simulink model "NarwhaleSimscape"  (R2021b)
settings: Solver=VariableStepAuto  StartTime=0.0  StopTime=12  FixedStep=10^-3  RelTol=1e-3
undefined symbols (not defined in the file): X, Y, Z
libraries: nesl_utility x34, sm_lib x28, slpidlib x5
(part 2 of 3)

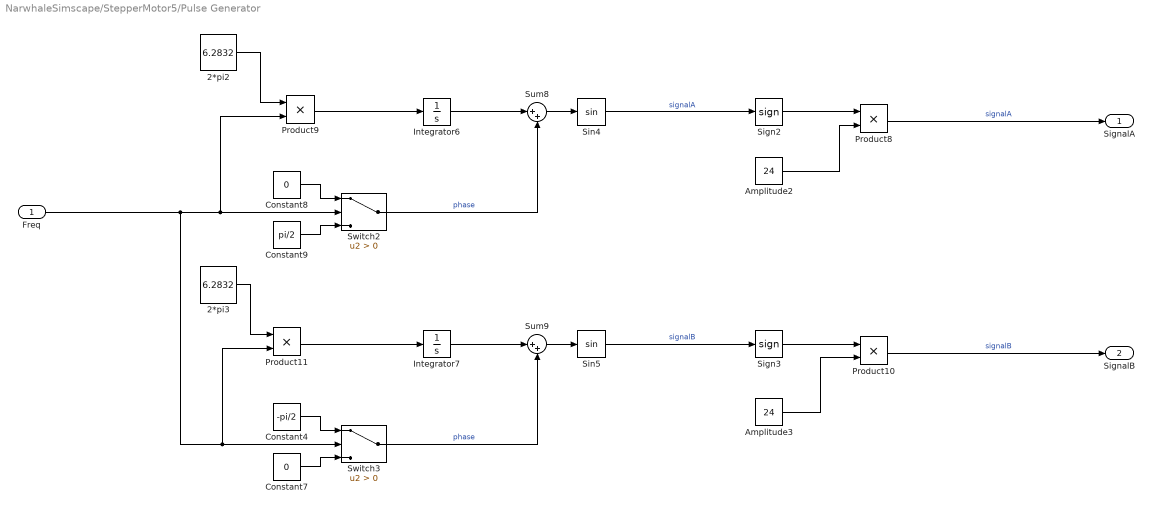
== system NarwhaleSimscape/StepperMotor5/Pulse Generator ==
  Freq : Inport
  2*pi2 : Constant  Value=6.2832
  2*pi3 : Constant  Value=6.2832
  Amplitude2 : Constant  Value=24
  Amplitude3 : Constant  Value=24
  Constant4 : Constant  Value=-pi/2
  Constant7 : Constant  Value=0
  Constant8 : Constant  Value=0
  Constant9 : Constant  Value=pi/2
  Integrator6 : Integrator
  Integrator7 : Integrator
  Product{8..11} (4 alike) : Product
  Sign2 : Signum
  Sign3 : Signum
  Sin4 : Trigonometry
  Sin5 : Trigonometry
  Sum8 : Sum  Inputs=|++
  Sum9 : Sum  Inputs=|++
  Switch2 : Switch  Criteria=u2 > Threshold
  Switch3 : Switch  Criteria=u2 > Threshold
  SignalA : Outport
  SignalB : Outport  Port=2
  wires:
  Product11/1 -> Integrator7/1
  Switch3/1 -> Sum9/2  "phase"
  Sum8/1 -> Sin4/1
  Sign3/1 -> Product10/1
  Integrator7/1 -> Sum9/1
  Freq/1 -> Product11/2, Switch3/2, Product9/2, Switch2/2
  Sin5/1 -> Sign3/1  "signalB"
  Sign2/1 -> Product8/1
  Product10/1 -> SignalB/1  "signalB"
  Product8/1 -> SignalA/1  "signalA"
  Amplitude3/1 -> Product10/2
  Sum9/1 -> Sin5/1
  Amplitude2/1 -> Product8/2
  Integrator6/1 -> Sum8/1
  Constant4/1 -> Switch3/1
  Constant7/1 -> Switch3/3
  2*pi3/1 -> Product11/1
  Switch2/1 -> Sum8/2  "phase"
  Constant9/1 -> Switch2/3
  Constant8/1 -> Switch2/1
  2*pi2/1 -> Product9/1
  Sin4/1 -> Sign2/1  "signalA"
  Product9/1 -> Integrator6/1

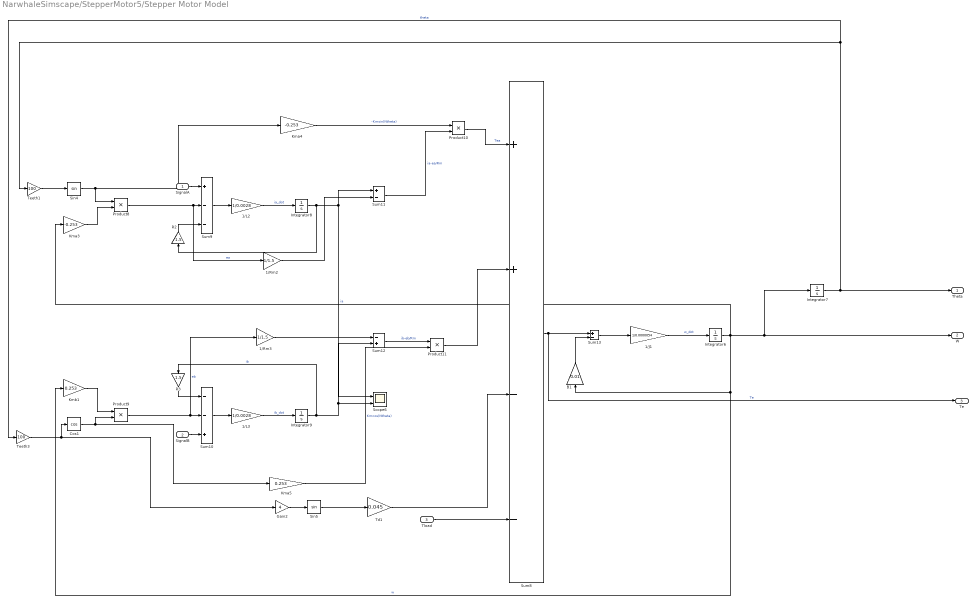
== system NarwhaleSimscape/StepperMotor5/Stepper Motor Model ==
  SignalA : Inport
  SignalB : Inport  Port=2
  Tload : Inport  Port=3
  1/J1 : Gain  Gain=1/0.0000054
  1/L2 : Gain  Gain=1/0.0028
  1/L3 : Gain  Gain=1/0.0028
  1/Rm2 : Gain  Gain=1/1.5
  1/Rm3 : Gain  Gain=1/1.5
  B1 : Gain  Gain=0.01
  Cos1 : Trigonometry  Operator=cos
  Gain2 : Gain  Gain=4
  Integrator{6..9} (4 alike) : Integrator
  Kma3 : Gain  Gain=-0.253
  Kma4 : Gain  Gain=-0.253
  Kma5 : Gain  Gain=0.253
  Kmb1 : Gain  Gain=0.253
  Product{8..11} (4 alike) : Product
  R2 : Gain  Gain=1.5
  R3 : Gain  Gain=1.5
  Scope6 : Scope  NumInputPorts=2
  Sin4 : Trigonometry
  Sin5 : Trigonometry
  Sum10 : Sum  Inputs=--+
  Sum11 : Sum  Inputs=+-
  Sum12 : Sum  Inputs=-+
  Sum13 : Sum  Inputs=+-
  Sum8 : Sum  Inputs=++--
  Sum9 : Sum  Inputs=+--
  Td1 : Gain  Gain=0.045
  Teeth1 : Gain  Gain=100
  Teeth3 : Gain  Gain=100
  Theta : Outport
  W : Outport  Port=2
  Te : Outport  Port=3
  wires:
  Sum10/1 -> 1/L3/1
  1/L3/1 -> Integrator9/1  "ib_dot"
  Cos1/1 -> Kma5/1, Product9/2
  Tload/1 -> Sum8/4
  Gain2/1 -> Sin5/1
  Sum9/1 -> 1/L2/1
  SignalB/1 -> Sum10/3
  Sum13/1 -> 1/J1/1
  Product8/1 -> 1/Rm2/1, Sum9/2  "ea"
  Product11/1 -> Sum8/2
  Teeth3/1 -> Gain2/1, Cos1/1
  SignalA/1 -> Sum9/1
  Sum11/1 -> Product10/2  "ia-ea/Rm"
  1/Rm3/1 -> Sum12/1
  B1/1 -> Sum13/2
  Integrator7/1 -> Theta/1, Teeth1/1, Teeth3/1  "theta"
  Integrator6/1 -> Kmb1/1, B1/1, Kma3/1, W/1, Integrator7/1  "w"
  Sin4/1 -> Kma4/1, Product8/1
  Integrator8/1 -> Scope6/1, Sum11/1, R2/1  "ia"
  R2/1 -> Sum9/3
  Product9/1 -> 1/Rm3/1, Sum10/2  "eb"
  Kma3/1 -> Product8/2
  Sum12/1 -> Product11/1  "ib-eb/Rm"
  1/Rm2/1 -> Sum11/2
  Kmb1/1 -> Product9/1
  Product10/1 -> Sum8/1  "Tea"
  Integrator9/1 -> Scope6/2, Sum12/2, R3/1  "ib"
  Sum8/1 -> Te/1, Sum13/1  "Te"
  1/J1/1 -> Integrator6/1  "w_dot"
  Kma4/1 -> Product10/1  "-Kmsin(Ntheta)"
  Sin5/1 -> Td1/1
  Kma5/1 -> Product11/2  "Kmcos(Ntheta)"
  1/L2/1 -> Integrator8/1  "ia_dot"
  Teeth1/1 -> Sin4/1
  R3/1 -> Sum10/1
  Td1/1 -> Sum8/3

== matlab function NarwhaleSimscape/NarWhale/MATLAB Function1 ==
  data: chi input; qbar output
function qbar  = IKnarwhale5(chi)
    h1= 275.99/1000; % lasted
    h2= 380/1000;
    l1= 20/1000;
    l2= 380/1000;
    l3= 268.23/1000;
    gammabar= [1 1 -1];
    q1 = atan2(gammabar(1)*chi(2),gammabar(1)*chi(1));
    % RRIK
    r = gammabar(2)*sqrt(chi(1)^2 + chi(2)^2)
    z24 = chi(3)+l3-h1
    x24 = r-l1
    if (sqrt(x24^2+z24^2)<= (l2+h2)) && (sqrt(x24^2+z24^2)>=(l2-h2))

        c2 = (x24^2+z24^2-h2^2-l2^2)/(2*h2*l2)
        s2 = gammabar(3)*sqrt(1-c2^2)
        q2 = (atan2(z24,x24)-atan2(l2*s2,h2+l2*c2))-(pi/2) 
        q3 = atan2(s2,c2)+(pi/2)
    else
        % สั่งเกินระยะแขน เกิดท่าประหลาด
        msg = 'error link range.';
        error(msg)
    end 
    q4 = -q2-q3;
    q5 = chi(4);
    qbar = [q1;q2;q3;q4;q5];
end

== matlab function NarwhaleSimscape/NarWhale/IVK_3chi_dot ==
  data: q input; qv5 input; qv output; chi_dot input
function qv = IVK(q,qv5,chi_dot) %q,qv5,chi_dot  % q,taskspace
% h1= 275.99/1000; % lasted
% h2= 380/1000;
% l1= 20.01/1000;
% l2= 380/1000;
% l3= 235/1000;
% h1= 275.99/1000; % lasted
h2= 380/1000;
l1= 20/1000;
l2= 380/1000;
l3= 268.23/1000;

% qv = [                                                                                                                                                                                                                                                                                                                                                                                                                                                                                                                                                                                                                                                                                                                                                                                                                                                                                                                                                                                                                                                                                                                                                                                                                                                                                                                                                                                                                                                                                                                                                                                                                                                                                                                                                                                                                                                                                                                                                                                                                                                                                                                                                                                                                                                                                                                                                                                                                                                                                                                                                                                                                                                                                                                                                                                                                                                                                                                                                                                                                                                                                                                                                                                                                                                                                                                                                                                                                                                                                                                                                                                                                                                                                                                                                                                                                                                                                                                                                                                                                                                                                                                                                                                                                                                                                                                                                                                                                                                                                                                                                                                                                                                                                                                                                                                                                                                                                                                                                                                                                                                                                                                                                                                                                                                                                                                                                                                                                                                                                                                                                                                                                                                                                                                                                                                                                                                                                                                                                                                                                                                                                                                                                                                                                                                                                                                                                                                                                                                                                                                                                                                                                                                                                       (taskspace(4)*cos(q(1)) - taskspace(3)*sin(q(1)))/(l1 + l2*cos(q(2) + q(3)) - 1.0*h2*sin(q(2)) + l3*sin(q(2) + q(3) + q(4)));
%                                                                                                                                                                                                                                                                                                                                                                                                                                                                                                                                                                                                                                                                                                                                                                                                                                                                                                                                                                                                                                                                                                                                                                                                                                                                                                                                                                                                                                                                                                                                                                                                                                                                                                                                                                                                                                                                                                                                                                                                                                                                                                                                                                                                                                                                                                                                                                                                                                                                                                                                                                                                                                                                                                                                                                                                                                                                                                                                                                                                                                                                                                                                                                     -(1.0*(l3^2*taskspace(2)*sin(q(2) + q(3) + q(4))^3*sin(q(2) + q(3))*sin(q(1))^3 + l1*taskspace(3)*cos(q(2) + q(3) + q(4))*cos(q(2) + q(3))*cos(q(1))^2 + l1*taskspace(5)*cos(q(2) + q(3) + q(4))*sin(q(2) + q(3))*cos(q(1))^3 + l2*taskspace(3)*cos(q(2) + q(3) + q(4))*cos(q(2) + q(3))^2*cos(q(1))^2 + l3*taskspace(3)*sin(q(2) + q(3) + q(4))^2*sin(q(2) + q(3))*sin(q(1))^2 + l1*l3*taskspace(1)*cos(q(2) + q(3) + q(4))^2*cos(q(2) + q(3))*sin(q(1))^2 - h2*taskspace(3)*cos(q(2) + q(3) + q(4))*cos(q(2) + q(3))*cos(q(1))^2*sin(q(2)) + l2*taskspace(4)*cos(q(2) + q(3) + q(4))*cos(q(2) + q(3))^2*cos(q(1))*sin(q(1)) + l3^2*taskspace(1)*cos(q(2) + q(3) + q(4))^2*sin(q(2) + q(3) + q(4))*cos(q(2) + q(3))*cos(q(1))^2 - h2*taskspace(5)*cos(q(2) + q(3) + q(4))*sin(q(2) + q(3))*cos(q(1))^3*sin(q(2)) + l1*taskspace(5)*cos(q(2) + q(3) + q(4))*sin(q(2) + q(3))*cos(q(1))*sin(q(1))^2 + l3^2*taskspace(1)*cos(q(2) + q(3) + q(4))*sin(q(2) + q(3) + q(4))^2*sin(q(2) + q(3))*cos(q(1))^2 + l3^2*taskspace(1)*cos(q(2) + q(3) + q(4))^2*sin(q(2) + q(3) + q(4))*cos(q(2) + q(3))*sin(q(1))^2 + l3^2*taskspace(2)*cos(q(2) + q(3) + q(4))*sin(q(2) + q(3) + q(4))^2*cos(q(2) + q(3))*sin(q(1))^3 + l1*l3*taskspace(2)*sin(q(2) + q(3) + q(4))^2*sin(q(2) + q(3))*sin(q(1))^3 - l3*taskspace(4)*sin(q(2) + q(3) + q(4))^2*sin(q(2) + q(3))*cos(q(1))*sin(q(1)) + l3^2*taskspace(1)*cos(q(2) + q(3) + q(4))*sin(q(2) + q(3) + q(4))^2*sin(q(2) + q(3))*sin(q(1))^2 + l3*taskspace(3)*cos(q(2) + q(3) + q(4))*sin(q(2) + q(3) + q(4))*cos(q(2) + q(3))*cos(q(1))^2 + l2*l3*taskspace(1)*cos(q(2) + q(3) + q(4))^2*cos(q(2) + q(3))^2*cos(q(1))^2 + l3*taskspace(3)*cos(q(2) + q(3) + q(4))*sin(q(2) + q(3) + q(4))*cos(q(2) + q(3))*sin(q(1))^2 + l3*taskspace(5)*cos(q(2) + q(3) + q(4))*sin(q(2) + q(3) + q(4))*sin(q(2) + q(3))*cos(q(1))^3 + l2*l3*taskspace(1)*cos(q(2) + q(3) + q(4))^2*cos(q(2) + q(3))^2*sin(q(1))^2 + l1*taskspace(4)*cos(q(2) + q(3) + q(4))*cos(q(2) + q(3))*cos(q(1))*sin(q(1)) + l2*taskspace(5)*cos(q(2) + q(3) + q(4))*cos(q(2) + q(3))*sin(q(2) + q(3))*cos(q(1))^3 + l3^2*taskspace(2)*sin(q(2) + q(3) + q(4))^3*sin(q(2) + q(3))*cos(q(1))^2*sin(q(1)) + l1*l3*taskspace(1)*cos(q(2) + q(3) + q(4))^2*cos(q(2) + q(3))*cos(q(1))^2 + l1*l3*taskspace(2)*sin(q(2) + q(3) + q(4))^2*sin(q(2) + q(3))*cos(q(1))^2*sin(q(1)) - h2*taskspace(5)*cos(q(2) + q(3) + q(4))*sin(q(2) + q(3))*cos(q(1))*sin(q(1))^2*sin(q(2)) - h2*l3*taskspace(2)*sin(q(2) + q(3) + q(4))^2*sin(q(2) + q(3))*sin(q(1))^3*sin(q(2)) + l2*l3*taskspace(2)*cos(q(2) + q(3) + q(4))*sin(q(2) + q(3) + q(4))*cos(q(2) + q(3))^2*sin(q(1))^3 + l3*taskspace(5)*cos(q(2) + q(3) + q(4))*sin(q(2) + q(3) + q(4))*sin(q(2) + q(3))*cos(q(1))*sin(q(1))^2 - h2*taskspace(4)*cos(q(2) + q(3) + q(4))*cos(q(2) + q(3))*cos(q(1))*sin(q(1))*sin(q(2)) + l2*taskspace(5)*cos(q(2) + q(3) + q(4))*cos(q(2) + q(3))*sin(q(2) + q(3))*cos(q(1))*sin(q(1))^2 + l2*l3*taskspace(2)*sin(q(2) + q(3) + q(4))^2*cos(q(2) + q(3))*sin(q(2) + q(3))*sin(q(1))^3 + l1*l3*taskspace(1)*cos(q(2) + q(3) + q(4))*sin(q(2) + q(3) + q(4))*sin(q(2) + q(3))*cos(q(1))^2 + l1*l3*taskspace(2)*cos(q(2) + q(3) + q(4))*sin(q(2) + q(3) + q(4))*cos(q(2) + q(3))*sin(q(1))^3 - h2*l3*taskspace(1)*cos(q(2) + q(3) + q(4))^2*cos(q(2) + q(3))*cos(q(1))^2*sin(q(2)) + l1*l3*taskspace(1)*cos(q(2) + q(3) + q(4))*sin(q(2) + q(3) + q(4))*sin(q(2) + q(3))*sin(q(1))^2 - h2*l3*taskspace(1)*cos(q(2) + q(3) + q(4))^2*cos(q(2) + q(3))*sin(q(1))^2*sin(q(2)) + l3^2*taskspace(2)*cos(q(2) + q(3) + q(4))*sin(q(2) + q(3) + q(4))^2*cos(q(2) + q(3))*cos(q(1))^2*sin(q(1)) + l2*l3*taskspace(2)*cos(q(2) + q(3) + q(4))*sin(q(2) + q(3) + q(4))*cos(q(2) + q(3))^2*cos(q(1))^2*sin(q(1)) + l2*l3*taskspace(1)*cos(q(2) + q(3) + q(4))*sin(q(2) + q(3) + q(4))*cos(q(2) + q(3))*sin(q(2) + q(3))*cos(q(1))^2 + l2*l3*taskspace(1)*cos(q(2) + q(3) + q(4))*sin(q(2) + q(3) + q(4))*cos(q(2) + q(3))*sin(q(2) + q(3))*sin(q(1))^2 + l2*l3*taskspace(2)*sin(q(2) + q(3) + q(4))^2*cos(q(2) + q(3))*sin(q(2) + q(3))*cos(q(1))^2*sin(q(1)) + l1*l3*taskspace(2)*cos(q(2) + q(3) + q(4))*sin(q(2) + q(3) + q(4))*cos(q(2) + q(3))*cos(q(1))^2*sin(q(1)) - h2*l3*taskspace(1)*cos(q(2) + q(3) + q(4))*sin(q(2) + q(3) + q(4))*sin(q(2) + q(3))*cos(q(1))^2*sin(q(2)) - h2*l3*taskspace(2)*cos(q(2) + q(3) + q(4))*sin(q(2) + q(3) + q(4))*cos(q(2) + q(3))*sin(q(1))^3*sin(q(2)) - h2*l3*taskspace(1)*cos(q(2) + q(3) + q(4))*sin(q(2) + q(3) + q(4))*sin(q(2) + q(3))*sin(q(1))^2*sin(q(2)) - h2*l3*taskspace(2)*sin(q(2) + q(3) + q(4))^2*sin(q(2) + q(3))*cos(q(1))^2*sin(q(1))*sin(q(2)) - h2*l3*taskspace(2)*cos(q(2) + q(3) + q(4))*sin(q(2) + q(3) + q(4))*cos(q(2) + q(3))*cos(q(1))^2*sin(q(1))*sin(q(2))))/(h2*cos(q(1))*cos(q(3))*(0.5*l3*sin(2*q(2) + 2*q(3) + 2*q(4)) + 0.5*l2*cos(2.0*q(2) + 2.0*q(3) + q(4)) + 0.5*h2*sin(q(3) + q(4)) - 0.5*h2*sin(2.0*q(2) + q(3) + q(4)) + 0.5*l2*cos(q(4)) + l1*cos(q(2) + q(3) + q(4))));
% (1.0*(h2^2*taskspace(3)*cos(q(2) + q(3) + q(4))*cos(q(1))^2*sin(q(2))^2 + l2^2*taskspace(3)*cos(q(2) + q(3) + q(4))*cos(q(2) + q(3))^2*cos(q(1))^2 + h2^2*l3*taskspace(1)*cos(q(2) + q(3) + q(4))^2*sin(q(1))^2*sin(q(2))^2 + l2*l3*taskspace(3)*sin(q(2) + q(3) + q(4))^2*sin(q(2) + q(3))*sin(q(1))^2 + l2^2*taskspace(5)*cos(q(2) + q(3) + q(4))*cos(q(2) + q(3))*sin(q(2) + q(3))*cos(q(1))^3 + h2*l3*taskspace(3)*sin(q(2) + q(3) + q(4))^2*cos(q(2))*sin(q(1))^2 + l2^2*taskspace(4)*cos(q(2) + q(3) + q(4))*cos(q(2) + q(3))^2*cos(q(1))*sin(q(1)) + l2*l3^2*taskspace(2)*sin(q(2) + q(3) + q(4))^3*sin(q(2) + q(3))*sin(q(1))^3 + l1*l2*taskspace(3)*cos(q(2) + q(3) + q(4))*cos(q(2) + q(3))*cos(q(1))^2 - 1.0*h2^2*taskspace(5)*cos(q(2) + q(3) + q(4))*cos(q(1))^3*cos(q(2))*sin(q(2)) + h2*l3^2*taskspace(2)*sin(q(2) + q(3) + q(4))^3*cos(q(2))*sin(q(1))^3 + l1*l2*taskspace(5)*cos(q(2) + q(3) + q(4))*sin(q(2) + q(3))*cos(q(1))^3 + h2^2*taskspace(4)*cos(q(2) + q(3) + q(4))*cos(q(1))*sin(q(1))*sin(q(2))^2 + l2^2*l3*taskspace(1)*cos(q(2) + q(3) + q(4))^2*cos(q(2) + q(3))^2*cos(q(1))^2 + h2*l1*taskspace(5)*cos(q(2) + q(3) + q(4))*cos(q(1))^3*cos(q(2)) + l2^2*l3*taskspace(1)*cos(q(2) + q(3) + q(4))^2*cos(q(2) + q(3))^2*sin(q(1))^2 - 1.0*h2*l1*taskspace(3)*cos(q(2) + q(3) + q(4))*cos(q(1))^2*sin(q(2)) + h2^2*l3*taskspace(1)*cos(q(2) + q(3) + q(4))^2*cos(q(1))^2*sin(q(2))^2 - 1.0*h2*l3*taskspace(3)*cos(q(2) + q(3) + q(4))*sin(q(2) + q(3) + q(4))*sin(q(1))^2*sin(q(2)) + l1*l2*taskspace(4)*cos(q(2) + q(3) + q(4))*cos(q(2) + q(3))*cos(q(1))*sin(q(1)) + l2^2*taskspace(5)*cos(q(2) + q(3) + q(4))*cos(q(2) + q(3))*sin(q(2) + q(3))*cos(q(1))*sin(q(1))^2 + l2^2*l3*taskspace(2)*sin(q(2) + q(3) + q(4))^2*cos(q(2) + q(3))*sin(q(2) + q(3))*sin(q(1))^3 - 1.0*h2*l1*taskspace(4)*cos(q(2) + q(3) + q(4))*cos(q(1))*sin(q(1))*sin(q(2)) + l2*l3^2*taskspace(2)*sin(q(2) + q(3) + q(4))^3*sin(q(2) + q(3))*cos(q(1))^2*sin(q(1)) + l1*l2*l3*taskspace(1)*cos(q(2) + q(3) + q(4))^2*cos(q(2) + q(3))*cos(q(1))^2 + h2*l2*taskspace(5)*cos(q(2) + q(3) + q(4))*cos(q(2) + q(3))*cos(q(1))^3*cos(q(2)) + l1*l2*l3*taskspace(1)*cos(q(2) + q(3) + q(4))^2*cos(q(2) + q(3))*sin(q(1))^2 + h2*l3^2*taskspace(2)*sin(q(2) + q(3) + q(4))^3*cos(q(1))^2*cos(q(2))*sin(q(1)) - 2.0*h2*l2*taskspace(3)*cos(q(2) + q(3) + q(4))*cos(q(2) + q(3))*cos(q(1))^2*sin(q(2)) + l2*l3^2*taskspace(1)*cos(q(2) + q(3) + q(4))^2*sin(q(2) + q(3) + q(4))*cos(q(2) + q(3))*cos(q(1))^2 - 1.0*h2^2*taskspace(5)*cos(q(2) + q(3) + q(4))*cos(q(1))*cos(q(2))*sin(q(1))^2*sin(q(2)) - 1.0*h2^2*l3*taskspace(2)*sin(q(2) + q(3) + q(4))^2*cos(q(2))*sin(q(1))^3*sin(q(2)) - 1.0*h2*l2*taskspace(5)*cos(q(2) + q(3) + q(4))*sin(q(2) + q(3))*cos(q(1))^3*sin(q(2)) + l1*l2*taskspace(5)*cos(q(2) + q(3) + q(4))*sin(q(2) + q(3))*cos(q(1))*sin(q(1))^2 + l2*l3^2*taskspace(1)*cos(q(2) + q(3) + q(4))*sin(q(2) + q(3) + q(4))^2*sin(q(2) + q(3))*cos(q(1))^2 + l2*l3^2*taskspace(1)*cos(q(2) + q(3) + q(4))^2*sin(q(2) + q(3) + q(4))*cos(q(2) + q(3))*sin(q(1))^2 + l2*l3^2*taskspace(2)*cos(q(2) + q(3) + q(4))*sin(q(2) + q(3) + q(4))^2*cos(q(2) + q(3))*sin(q(1))^3 + l2^2*l3*taskspace(2)*cos(q(2) + q(3) + q(4))*sin(q(2) + q(3) + q(4))*cos(q(2) + q(3))^2*sin(q(1))^3 + l1*l2*l3*taskspace(2)*sin(q(2) + q(3) + q(4))^2*sin(q(2) + q(3))*sin(q(1))^3 - 1.0*l2*l3*taskspace(4)*sin(q(2) + q(3) + q(4))^2*sin(q(2) + q(3))*cos(q(1))*sin(q(1)) + l2*l3^2*taskspace(1)*cos(q(2) + q(3) + q(4))*sin(q(2) + q(3) + q(4))^2*sin(q(2) + q(3))*sin(q(1))^2 - 1.0*h2*l1*l3*taskspace(1)*cos(q(2) + q(3) + q(4))^2*cos(q(1))^2*sin(q(2)) + h2*l1*taskspace(5)*cos(q(2) + q(3) + q(4))*cos(q(1))*cos(q(2))*sin(q(1))^2 + h2*l3^2*taskspace(1)*cos(q(2) + q(3) + q(4))*sin(q(2) + q(3) + q(4))^2*cos(q(1))^2*cos(q(2)) - 1.0*h2*l1*l3*taskspace(1)*cos(q(2) + q(3) + q(4))^2*sin(q(1))^2*sin(q(2)) + h2*l1*l3*taskspace(2)*sin(q(2) + q(3) + q(4))^2*cos(q(2))*sin(q(1))^3 - 1.0*h2*l3*taskspace(4)*sin(q(2) + q(3) + q(4))^2*cos(q(1))*cos(q(2))*sin(q(1)) + h2*l3^2*taskspace(1)*cos(q(2) + q(3) + q(4))*sin(q(2) + q(3) + q(4))^2*cos(q(2))*sin(q(1))^2 - 1.0*h2*l3^2*taskspace(1)*cos(q(2) + q(3) + q(4))^2*sin(q(2) + q(3) + q(4))*cos(q(1))^2*sin(q(2)) + l2*l3*taskspace(3)*cos(q(2) + q(3) + q(4))*sin(q(2) + q(3) + q(4))*cos(q(2) + q(3))*cos(q(1))^2 - 1.0*h2*l3^2*taskspace(1)*cos(q(2) + q(3) + q(4))^2*sin(q(2) + q(3) + q(4))*sin(q(1))^2*sin(q(2)) - 1.0*h2*l3^2*taskspace(2)*cos(q(2) + q(3) + q(4))*sin(q(2) + q(3) + q(4))^2*sin(q(1))^3*sin(q(2)) + h2^2*l3*taskspace(2)*cos(q(2) + q(3) + q(4))*sin(q(2) + q(3) + q(4))*sin(q(1))^3*sin(q(2))^2 + l2*l3*taskspace(3)*cos(q(2) + q(3) + q(4))*sin(q(2) + q(3) + q(4))*cos(q(2) + q(3))*sin(q(1))^2 + l2*l3*taskspace(5)*cos(q(2) + q(3) + q(4))*sin(q(2) + q(3) + q(4))*sin(q(2) + q(3))*cos(q(1))^3 + h2*l3*taskspace(5)*cos(q(2) + q(3) + q(4))*sin(q(2) + q(3) + q(4))*cos(q(1))^3*cos(q(2)) - 1.0*h2*l3*taskspace(3)*cos(q(2) + q(3) + q(4))*sin(q(2) + q(3) + q(4))*cos(q(1))^2*sin(q(2)) - 2.0*h2*l2*taskspace(4)*cos(q(2) + q(3) + q(4))*cos(q(2) + q(3))*cos(q(1))*sin(q(1))*sin(q(2)) + l2^2*l3*taskspace(2)*sin(q(2) + q(3) + q(4))^2*cos(q(2) + q(3))*sin(q(2) + q(3))*cos(q(1))^2*sin(q(1)) - 1.0*h2^2*l3*taskspace(1)*cos(q(2) + q(3) + q(4))*sin(q(2) + q(3) + q(4))*cos(q(1))^2*cos(q(2))*sin(q(2)) + l1*l2*l3*taskspace(1)*cos(q(2) + q(3) + q(4))*sin(q(2) + q(3) + q(4))*sin(q(2) + q(3))*cos(q(1))^2 + l1*l2*l3*taskspace(2)*cos(q(2) + q(3) + q(4))*sin(q(2) + q(3) + q(4))*cos(q(2) + q(3))*sin(q(1))^3 - 1.0*h2^2*l3*taskspace(1)*cos(q(2) + q(3) + q(4))*sin(q(2) + q(3) + q(4))*cos(q(2))*sin(q(1))^2*sin(q(2)) - 2.0*h2*l2*l3*taskspace(1)*cos(q(2) + q(3) + q(4))^2*cos(q(2) + q(3))*cos(q(1))^2*sin(q(2)) + l1*l2*l3*taskspace(1)*cos(q(2) + q(3) + q(4))*sin(q(2) + q(3) + q(4))*sin(q(2) + q(3))*sin(q(1))^2 + h2*l2*taskspace(5)*cos(q(2) + q(3) + q(4))*cos(q(2) + q(3))*cos(q(1))*cos(q(2))*sin(q(1))^2 - 2.0*h2*l2*l3*taskspace(1)*cos(q(2) + q(3) + q(4))^2*cos(q(2) + q(3))*sin(q(1))^2*sin(q(2)) + h2*l2*l3*taskspace(2)*sin(q(2) + q(3) + q(4))^2*cos(q(2) + q(3))*cos(q(2))*sin(q(1))^3 + h2*l1*l3*taskspace(1)*cos(q(2) + q(3) + q(4))*sin(q(2) + q(3) + q(4))*cos(q(1))^2*cos(q(2)) - 1.0*h2^2*l3*taskspace(2)*sin(q(2) + q(3) + q(4))^2*cos(q(1))^2*cos(q(2))*sin(q(1))*sin(q(2)) + l2*l3^2*taskspace(2)*cos(q(2) + q(3) + q(4))*sin(q(2) + q(3) + q(4))^2*cos(q(2) + q(3))*cos(q(1))^2*sin(q(1)) + l2^2*l3*taskspace(2)*cos(q(2) + q(3) + q(4))*sin(q(2) + q(3) + q(4))*cos(q(2) + q(3))^2*cos(q(1))^2*sin(q(1)) + h2*l1*l3*taskspace(1)*cos(q(2) + q(3) + q(4))*sin(q(2) + q(3) + q(4))*cos(q(2))*sin(q(1))^2 + l1*l2*l3*taskspace(2)*sin(q(2) + q(3) + q(4))^2*sin(q(2) + q(3))*cos(q(1))^2*sin(q(1)) - 1.0*h2*l2*taskspace(5)*cos(q(2) + q(3) + q(4))*sin(q(2) + q(3))*cos(q(1))*sin(q(1))^2*sin(q(2)) - 1.0*h2*l2*l3*taskspace(2)*sin(q(2) + q(3) + q(4))^2*sin(q(2) + q(3))*sin(q(1))^3*sin(q(2)) - 1.0*h2*l1*l3*taskspace(2)*cos(q(2) + q(3) + q(4))*sin(q(2) + q(3) + q(4))*sin(q(1))^3*sin(q(2)) + h2*l1*l3*taskspace(2)*sin(q(2) + q(3) + q(4))^2*cos(q(1))^2*cos(q(2))*sin(q(1)) - 1.0*h2*l3^2*taskspace(2)*cos(q(2) + q(3) + q(4))*sin(q(2) + q(3) + q(4))^2*cos(q(1))^2*sin(q(1))*sin(q(2)) + h2^2*l3*taskspace(2)*cos(q(2) + q(3) + q(4))*sin(q(2) + q(3) + q(4))*cos(q(1))^2*sin(q(1))*sin(q(2))^2 + l2*l3*taskspace(5)*cos(q(2) + q(3) + q(4))*sin(q(2) + q(3) + q(4))*sin(q(2) + q(3))*cos(q(1))*sin(q(1))^2 + h2*l3*taskspace(5)*cos(q(2) + q(3) + q(4))*sin(q(2) + q(3) + q(4))*cos(q(1))*cos(q(2))*sin(q(1))^2 + l2^2*l3*taskspace(1)*cos(q(2) + q(3) + q(4))*sin(q(2) + q(3) + q(4))*cos(q(2) + q(3))*sin(q(2) + q(3))*cos(q(1))^2 + l2^2*l3*taskspace(1)*cos(q(2) + q(3) + q(4))*sin(q(2) + q(3) + q(4))*cos(q(2) + q(3))*sin(q(2) + q(3))*sin(q(1))^2 + h2*l2*l3*taskspace(1)*cos(q(2) + q(3) + q(4))*sin(q(2) + q(3) + q(4))*cos(q(2) + q(3))*cos(q(2))*sin(q(1))^2 + l1*l2*l3*taskspace(2)*cos(q(2) + q(3) + q(4))*sin(q(2) + q(3) + q(4))*cos(q(2) + q(3))*cos(q(1))^2*sin(q(1)) - 1.0*h2*l2*l3*taskspace(1)*cos(q(2) + q(3) + q(4))*sin(q(2) + q(3) + q(4))*sin(q(2) + q(3))*cos(q(1))^2*sin(q(2)) - 2.0*h2*l2*l3*taskspace(2)*cos(q(2) + q(3) + q(4))*sin(q(2) + q(3) + q(4))*cos(q(2) + q(3))*sin(q(1))^3*sin(q(2)) + h2*l2*l3*taskspace(2)*sin(q(2) + q(3) + q(4))^2*cos(q(2) + q(3))*cos(q(1))^2*cos(q(2))*sin(q(1)) - 1.0*h2*l2*l3*taskspace(1)*cos(q(2) + q(3) + q(4))*sin(q(2) + q(3) + q(4))*sin(q(2) + q(3))*sin(q(1))^2*sin(q(2)) - 1.0*h2*l2*l3*taskspace(2)*sin(q(2) + q(3) + q(4))^2*sin(q(2) + q(3))*cos(q(1))^2*sin(q(1))*sin(q(2)) - 1.0*h2*l1*l3*taskspace(2)*cos(q(2) + q(3) + q(4))*sin(q(2) + q(3) + q(4))*cos(q(1))^2*sin(q(1))*sin(q(2)) + h2*l2*l3*taskspace(1)*cos(q(2) + q(3) + q(4))*sin(q(2) + q(3) + q(4))*cos(q(2) + q(3))*cos(q(1))^2*cos(q(2)) - 2.0*h2*l2*l3*taskspace(2)*cos(q(2) + q(3) + q(4))*sin(q(2) + q(3) + q(4))*cos(q(2) + q(3))*cos(q(1))^2*sin(q(1))*sin(q(2))))/(h2*l2*cos(q(1))*cos(q(3))*(0.5*l3*sin(2*q(2) + 2*q(3) + 2*q(4)) + 0.5*l2*cos(2.0*q(2) + 2.0*q(3) + q(4)) + 0.5*h2*sin(q(3) + q(4)) - 0.5*h2*sin(2.0*q(2) + q(3) + q(4)) + 0.5*l2*cos(q(4)) + l1*cos(q(2) + q(3) + q(4))));
%                                                                                                                                                                                                                                                                                                                                                                                                                                                                                                                                                                                                                                                                                                                                                                                                                                                                                                                                                                                                                                                                                                                                                                                     -(1.0*(l3^2*taskspace(2)*sin(q(2) + q(3) + q(4))^3*cos(q(2))*sin(q(1))^3 + l1*taskspace(5)*cos(q(2) + q(3) + q(4))*cos(q(1))^3*cos(q(2)) - l1*taskspace(3)*cos(q(2) + q(3) + q(4))*cos(q(1))^2*sin(q(2)) + h2*taskspace(3)*cos(q(2) + q(3) + q(4))*cos(q(1))^2*sin(q(2))^2 + l3*taskspace(3)*sin(q(2) + q(3) + q(4))^2*cos(q(2))*sin(q(1))^2 + l2*taskspace(5)*cos(q(2) + q(3) + q(4))*cos(q(2) + q(3))*cos(q(1))^3*cos(q(2)) + l3^2*taskspace(2)*sin(q(2) + q(3) + q(4))^3*cos(q(1))^2*cos(q(2))*sin(q(1)) - l2*taskspace(3)*cos(q(2) + q(3) + q(4))*cos(q(2) + q(3))*cos(q(1))^2*sin(q(2)) + l2*taskspace(3)*sin(q(2) + q(3) + q(4))*cos(q(2) + q(3))*cos(q(2))*sin(q(1))^2 - l1*l3*taskspace(1)*cos(q(2) + q(3) + q(4))^2*cos(q(1))^2*sin(q(2)) - h2*taskspace(5)*cos(q(2) + q(3) + q(4))*cos(q(1))^3*cos(q(2))*sin(q(2)) + l1*taskspace(5)*cos(q(2) + q(3) + q(4))*cos(q(1))*cos(q(2))*sin(q(1))^2 + l2*taskspace(3)*sin(q(2) + q(3) + q(4))*sin(q(2) + q(3))*sin(q(1))^2*sin(q(2)) + l3^2*taskspace(1)*cos(q(2) + q(3) + q(4))*sin(q(2) + q(3) + q(4))^2*cos(q(1))^2*cos(q(2)) - l1*l3*taskspace(1)*cos(q(2) + q(3) + q(4))^2*sin(q(1))^2*sin(q(2)) + l1*l3*taskspace(2)*sin(q(2) + q(3) + q(4))^2*cos(q(2))*sin(q(1))^3 + h2*taskspace(4)*cos(q(2) + q(3) + q(4))*cos(q(1))*sin(q(1))*sin(q(2))^2 - l3*taskspace(4)*sin(q(2) + q(3) + q(4))^2*cos(q(1))*cos(q(2))*sin(q(1)) + l3^2*taskspace(1)*cos(q(2) + q(3) + q(4))*sin(q(2) + q(3) + q(4))^2*cos(q(2))*sin(q(1))^2 - l3^2*taskspace(1)*cos(q(2) + q(3) + q(4))^2*sin(q(2) + q(3) + q(4))*cos(q(1))^2*sin(q(2)) - l3^2*taskspace(1)*cos(q(2) + q(3) + q(4))^2*sin(q(2) + q(3) + q(4))*sin(q(1))^2*sin(q(2)) - l3^2*taskspace(2)*cos(q(2) + q(3) + q(4))*sin(q(2) + q(3) + q(4))^2*sin(q(1))^3*sin(q(2)) + l3*taskspace(5)*cos(q(2) + q(3) + q(4))*sin(q(2) + q(3) + q(4))*cos(q(1))^3*cos(q(2)) - l3*taskspace(3)*cos(q(2) + q(3) + q(4))*sin(q(2) + q(3) + q(4))*cos(q(1))^2*sin(q(2)) + h2*l3*taskspace(1)*cos(q(2) + q(3) + q(4))^2*cos(q(1))^2*sin(q(2))^2 - l3*taskspace(3)*cos(q(2) + q(3) + q(4))*sin(q(2) + q(3) + q(4))*sin(q(1))^2*sin(q(2)) + h2*l3*taskspace(1)*cos(q(2) + q(3) + q(4))^2*sin(q(1))^2*sin(q(2))^2 + l2^2*taskspace(1)*cos(q(2) + q(3) + q(4))*cos(q(2) + q(3))^2*cos(q(1))^2*cos(q(2)) + l2^2*taskspace(1)*cos(q(2) + q(3) + q(4))*cos(q(2) + q(3))^2*cos(q(2))*sin(q(1))^2 + l2^2*taskspace(2)*sin(q(2) + q(3) + q(4))*cos(q(2) + q(3))^2*cos(q(2))*sin(q(1))^3 - l1*taskspace(4)*cos(q(2) + q(3) + q(4))*cos(q(1))*sin(q(1))*sin(q(2)) + l1*l3*taskspace(1)*cos(q(2) + q(3) + q(4))*sin(q(2) + q(3) + q(4))*cos(q(2))*sin(q(1))^2 - h2*l2*taskspace(2)*sin(q(2) + q(3) + q(4))*sin(q(2) + q(3))*sin(q(1))^3*sin(q(2))^2 + l2*l3*taskspace(2)*sin(q(2) + q(3) + q(4))^2*sin(q(2) + q(3))*sin(q(1))^3*sin(q(2)) - l1*l3*taskspace(2)*cos(q(2) + q(3) + q(4))*sin(q(2) + q(3) + q(4))*sin(q(1))^3*sin(q(2)) + l1*l3*taskspace(2)*sin(q(2) + q(3) + q(4))^2*cos(q(1))^2*cos(q(2))*sin(q(1)) - h2*taskspace(5)*cos(q(2) + q(3) + q(4))*cos(q(1))*cos(q(2))*sin(q(1))^2*sin(q(2)) + l2^2*taskspace(1)*cos(q(2) + q(3) + q(4))*cos(q(2) + q(3))*sin(q(2) + q(3))*cos(q(1))^2*sin(q(2)) - h2*l3*taskspace(2)*sin(q(2) + q(3) + q(4))^2*cos(q(2))*sin(q(1))^3*sin(q(2)) + l2^2*taskspace(1)*cos(q(2) + q(3) + q(4))*cos(q(2) + q(3))*sin(q(2) + q(3))*sin(q(1))^2*sin(q(2)) - l3^2*taskspace(2)*cos(q(2) + q(3) + q(4))*sin(q(2) + q(3) + q(4))^2*cos(q(1))^2*sin(q(1))*sin(q(2)) + l2^2*taskspace(2)*sin(q(2) + q(3) + q(4))*cos(q(2) + q(3))*sin(q(2) + q(3))*sin(q(1))^3*sin(q(2)) + l3*taskspace(5)*cos(q(2) + q(3) + q(4))*sin(q(2) + q(3) + q(4))*cos(q(1))*cos(q(2))*sin(q(1))^2 + h2*l3*taskspace(2)*cos(q(2) + q(3) + q(4))*sin(q(2) + q(3) + q(4))*sin(q(1))^3*sin(q(2))^2 + l1*l2*taskspace(1)*cos(q(2) + q(3) + q(4))*cos(q(2) + q(3))*cos(q(1))^2*cos(q(2)) + l1*l2*taskspace(1)*cos(q(2) + q(3) + q(4))*cos(q(2) + q(3))*cos(q(2))*sin(q(1))^2 + l1*l2*taskspace(1)*cos(q(2) + q(3) + q(4))*sin(q(2) + q(3))*cos(q(1))^2*sin(q(2)) + l1*l2*taskspace(2)*sin(q(2) + q(3) + q(4))*cos(q(2) + q(3))*cos(q(2))*sin(q(1))^3 - l2*taskspace(4)*cos(q(2) + q(3) + q(4))*cos(q(2) + q(3))*cos(q(1))*sin(q(1))*sin(q(2)) - l2*taskspace(4)*sin(q(2) + q(3) + q(4))*cos(q(2) + q(3))*cos(q(1))*cos(q(2))*sin(q(1)) + l1*l2*taskspace(1)*cos(q(2) + q(3) + q(4))*sin(q(2) + q(3))*sin(q(1))^2*sin(q(2)) + l1*l2*taskspace(2)*sin(q(2) + q(3) + q(4))*sin(q(2) + q(3))*sin(q(1))^3*sin(q(2)) + l2^2*taskspace(2)*sin(q(2) + q(3) + q(4))*cos(q(2) + q(3))^2*cos(q(1))^2*cos(q(2))*sin(q(1)) - l2*taskspace(4)*sin(q(2) + q(3) + q(4))*sin(q(2) + q(3))*cos(q(1))*sin(q(1))*sin(q(2)) - l2*l3*taskspace(1)*cos(q(2) + q(3) + q(4))^2*cos(q(2) + q(3))*cos(q(1))^2*sin(q(2)) + l2*taskspace(5)*cos(q(2) + q(3) + q(4))*cos(q(2) + q(3))*cos(q(1))*cos(q(2))*sin(q(1))^2 - h2*l2*taskspace(1)*cos(q(2) + q(3) + q(4))*sin(q(2) + q(3))*cos(q(1))^2*sin(q(2))^2 - l2*l3*taskspace(1)*cos(q(2) + q(3) + q(4))^2*cos(q(2) + q(3))*sin(q(1))^2*sin(q(2)) + 2.0*l2*l3*taskspace(2)*sin(q(2) + q(3) + q(4))^2*cos(q(2) + q(3))*cos(q(2))*sin(q(1))^3 + l1*l3*taskspace(1)*cos(q(2) + q(3) + q(4))*sin(q(2) + q(3) + q(4))*cos(q(1))^2*cos(q(2)) - h2*l2*taskspace(1)*cos(q(2) + q(3) + q(4))*sin(q(2) + q(3))*sin(q(1))^2*sin(q(2))^2 - h2*l3*taskspace(2)*sin(q(2) + q(3) + q(4))^2*cos(q(1))^2*cos(q(2))*sin(q(1))*sin(q(2)) + l2^2*taskspace(2)*sin(q(2) + q(3) + q(4))*cos(q(2) + q(3))*sin(q(2) + q(3))*cos(q(1))^2*sin(q(1))*sin(q(2)) + h2*l3*taskspace(2)*cos(q(2) + q(3) + q(4))*sin(q(2) + q(3) + q(4))*cos(q(1))^2*sin(q(1))*sin(q(2))^2 - h2*l2*taskspace(1)*cos(q(2) + q(3) + q(4))*cos(q(2) + q(3))*cos(q(1))^2*cos(q(2))*sin(q(2)) - h2*l2*taskspace(1)*cos(q(2) + q(3) + q(4))*cos(q(2) + q(3))*cos(q(2))*sin(q(1))^2*sin(q(2)) + l1*l2*taskspace(2)*sin(q(2) + q(3) + q(4))*cos(q(2) + q(3))*cos(q(1))^2*cos(q(2))*sin(q(1)) - h2*l2*taskspace(2)*sin(q(2) + q(3) + q(4))*cos(q(2) + q(3))*cos(q(2))*sin(q(1))^3*sin(q(2)) + l1*l2*taskspace(2)*sin(q(2) + q(3) + q(4))*sin(q(2) + q(3))*cos(q(1))^2*sin(q(1))*sin(q(2)) + 2.0*l2*l3*taskspace(1)*cos(q(2) + q(3) + q(4))*sin(q(2) + q(3) + q(4))*cos(q(2) + q(3))*cos(q(1))^2*cos(q(2)) + 2.0*l2*l3*taskspace(1)*cos(q(2) + q(3) + q(4))*sin(q(2) + q(3) + q(4))*cos(q(2) + q(3))*cos(q(2))*sin(q(1))^2 + l2*l3*taskspace(1)*cos(q(2) + q(3) + q(4))*sin(q(2) + q(3) + q(4))*sin(q(2) + q(3))*cos(q(1))^2*sin(q(2)) - l2*l3*taskspace(2)*cos(q(2) + q(3) + q(4))*sin(q(2) + q(3) + q(4))*cos(q(2) + q(3))*sin(q(1))^3*sin(q(2)) + 2.0*l2*l3*taskspace(2)*sin(q(2) + q(3) + q(4))^2*cos(q(2) + q(3))*cos(q(1))^2*cos(q(2))*sin(q(1)) + l2*l3*taskspace(1)*cos(q(2) + q(3) + q(4))*sin(q(2) + q(3) + q(4))*sin(q(2) + q(3))*sin(q(1))^2*sin(q(2)) - h2*l3*taskspace(1)*cos(q(2) + q(3) + q(4))*sin(q(2) + q(3) + q(4))*cos(q(1))^2*cos(q(2))*sin(q(2)) - h2*l2*taskspace(2)*sin(q(2) + q(3) + q(4))*sin(q(2) + q(3))*cos(q(1))^2*sin(q(1))*sin(q(2))^2 - h2*l3*taskspace(1)*cos(q(2) + q(3) + q(4))*sin(q(2) + q(3) + q(4))*cos(q(2))*sin(q(1))^2*sin(q(2)) + l2*l3*taskspace(2)*sin(q(2) + q(3) + q(4))^2*sin(q(2) + q(3))*cos(q(1))^2*sin(q(1))*sin(q(2)) - l1*l3*taskspace(2)*cos(q(2) + q(3) + q(4))*sin(q(2) + q(3) + q(4))*cos(q(1))^2*sin(q(1))*sin(q(2)) - h2*l2*taskspace(2)*sin(q(2) + q(3) + q(4))*cos(q(2) + q(3))*cos(q(1))^2*cos(q(2))*sin(q(1))*sin(q(2)) - l2*l3*taskspace(2)*cos(q(2) + q(3) + q(4))*sin(q(2) + q(3) + q(4))*cos(q(2) + q(3))*cos(q(1))^2*sin(q(1))*sin(q(2))))/(l2*cos(q(1))*cos(q(3))*(0.5*l3*sin(2*q(2) + 2*q(3) + 2*q(4)) + 0.5*l2*cos(2.0*q(2) + 2.0*q(3) + q(4)) + 0.5*h2*sin(q(3) + q(4)) - 0.5*h2*sin(2.0*q(2) + q(3) + q(4)) + 0.5*l2*cos(q(4)) + l1*cos(q(2) + q(3) + q(4))));
%                                                                                                                                                                                                                                                                                                                                                                                                                                                                                                                                                                                                                                                                                                                                                                                                                                                                                                                                                                                                                                                                                                                                                                                                                                                                                                                                                                                                                                                                                                                                                                                                                                                                                                                                                                                                                                                                                                                                                                                                                                                                                                                                                                                                                                                                                                                                                                                                                                                                                                                                                                                                                                                                                                                                                                                                                                                                                                                                                                                                                                                                                                                                                                                                                                                                                                                                                                                                                                                                                                                                                                                                                                                                                                                                                                                                                                                                                                                                                                                                                                                                                                                                                                                                                                                                                                                                                                                                                                                                                                                                                                                                                                                                                                                                                                                                                                                                                                                                                                                                                                                                                                                                                                                                                                                                                                                                                                                                                                                                                                                                                                                                                                                                                                                                                                                                                                                                                                                                                                                                                                                                                                                                                                                                                                                                                                                                                                                                                                                                                               -(1.0*(l1*taskspace(2) - 1.0*taskspace(4)*cos(q(1)) + taskspace(3)*sin(q(1)) - 1.0*h2*taskspace(2)*sin(q(2)) + 1.0*l3*taskspace(2)*sin(q(2) + q(3) + q(4)) + 1.0*l2*taskspace(2)*cos(q(2) + q(3))))/(0.5*l3*sin(2*q(2) + 2*q(3) + 2*q(4)) - 0.5*h2*sin(2*q(2) + q(3) + q(4)) + 0.5*h2*sin(q(3) + q(4)) + 0.5*l2*cos(q(4)) + 0.5*l2*cos(2*q(2) + 2*q(3) + q(4)) + 1.0*l1*cos(q(2) + q(3) + q(4)))]
%  
% 
%Jv5 ตรงแล้ว
Jv4 =[ -sin(q(1))*(l1 + l2*cos(q(2) + q(3)) - h2*sin(q(2))), -cos(q(1))*(l2*sin(q(2) + q(3)) + h2*cos(q(2))), -l2*sin(q(2) + q(3))*cos(q(1));
        cos(q(1))*(l1 + l2*cos(q(2) + q(3)) - h2*sin(q(2))), -sin(q(1))*(l2*sin(q(2) + q(3)) + h2*cos(q(2))), -l2*sin(q(2) + q(3))*sin(q(1));
                                                  0,            l2*cos(q(2) + q(3)) - h2*sin(q(2)),          l2*cos(q(2) + q(3))]

% Jv52 = [                                                   1,                                               0,                              0,       -1;
%         -sin(q(1))*(l1 + l2*cos(q(2) + q(3)) - h2*sin(q(2))), -cos(q(1))*(l2*sin(q(2) + q(3)) + h2*cos(q(2))), -l2*sin(q(2) + q(3))*cos(q(1)),        0;
%          cos(q(1))*(l1 + l2*cos(q(2) + q(3)) - h2*sin(q(2))), -sin(q(1))*(l2*sin(q(2) + q(3)) + h2*cos(q(2))), -l2*sin(q(2) + q(3))*sin(q(1)),        0;
%                                                            0,              l2*cos(q(2) + q(3)) - h2*sin(q(2)),            l2*cos(q(2) + q(3)),        0]
%Jv52 ไม่ตรง
% Jev3 = [- sin(q(1))*(l1 + l2*cos(q(2) + q(3)) - h2*sin(q(2))) , l3*cos(q(1)) - cos(q(1))*(l2*sin(q(2) + q(3)) + h2*cos(q(2))), -cos(q(1))*(l2*sin(q(2) + q(3)) - l3);
%    cos(q(1))*(l1 + l2*cos(q(2) + q(3)) - h2*sin(q(2)))        , l3*sin(q(1)) - sin(q(1))*(l2*sin(q(2) + q(3)) + h2*cos(q(2))), -sin(q(1))*(l2*sin(q(2) + q(3)) - l3);
%                                                            0  ,  l2*cos(q(2) + q(3)) - h2*sin(q(2))                          ,  l2*cos(q(2) + q(3)) ];
%jev3 ไม่ถูก
% Jev4=[                                                     1,                                                             0,                                     0,                 -1;
%       - sin(q(1))*(l1 + l2*cos(q(2) + q(3)) - h2*sin(q(2))) , l3*cos(q(1)) - cos(q(1))*(l2*sin(q(2) + q(3)) + h2*cos(q(2))), -cos(q(1))*(l2*sin(q(2) + q(3)) - l3),                  0;
%         cos(q(1))*(l1 + l2*cos(q(2) + q(3)) - h2*sin(q(2))) , l3*sin(q(1)) - sin(q(1))*(l2*sin(q(2) + q(3)) + h2*cos(q(2))), -sin(q(1))*(l2*sin(q(2) + q(3)) - l3),                  0;
%                                                            0,                           l2*cos(q(2) + q(3)) - h2*sin(q(2)) ,                  l2*cos(q(2) + q(3)) ,                  0] 
% jev4 ไม่ตรงเลย
% q1 =q(1)
% q2=q(2)
% q3=q(3)
% q4 = -q2-q3
% Je =  [- sin(q1)*(l1 + l2*cos(q2 + q3) - h2*sin(q2)) - l3*sin(q2 + q3 + q4)*sin(q1), l3*cos(q2 + q3 + q4)*cos(q1) - cos(q1)*(l2*sin(q2 + q3) + h2*cos(q2)), -cos(q1)*(l2*sin(q2 + q3) - l3*cos(q2 + q3 + q4));
%   cos(q1)*(l1 + l2*cos(q2 + q3) - h2*sin(q2)) + l3*sin(q2 + q3 + q4)*cos(q1), l3*cos(q2 + q3 + q4)*sin(q1) - sin(q1)*(l2*sin(q2 + q3) + h2*cos(q2)), -sin(q1)*(l2*sin(q2 + q3) - l3*cos(q2 + q3 + q4));
%                                                                            0,                   l2*cos(q2 + q3) - h2*sin(q2) + l3*sin(q2 + q3 + q4),            l2*cos(q2 + q3) + l3*sin(q2 + q3 + q4)]
%  
% Je =[                                      0,                                      sin(q1),                        sin(q1),    sin(q1),  0;
%                                            0,                                     -cos(q1),                       -cos(q1),   -cos(q1),  0;
%                                            1,                                            0,                              0,          0, -1;
% -sin(q1)*(l1 + l2*cos(q2 + q3) - h2*sin(q2)), -cos(q1)*(l2*sin(q2 + q3) - l3 + h2*cos(q2)), cos(q1)*(l3 - l2*sin(q2 + q3)), l3*cos(q1),  0;
%  cos(q1)*(l1 + l2*cos(q2 + q3) - h2*sin(q2)), -sin(q1)*(l2*sin(q2 + q3) - l3 + h2*cos(q2)), sin(q1)*(l3 - l2*sin(q2 + q3)), l3*sin(q1),  0;
%                                            0,                 l2*cos(q2 + q3) - h2*sin(q2),                l2*cos(q2 + q3),          0,  0] 

qvbar = Jv4 \ chi_dot
qv = [qvbar(1); qvbar(2); qvbar(3); -qvbar(2)-qvbar(3); qv5]

end

== matlab function NarwhaleSimscape/NarWhale/MATLAB Function2 ==
  data: rotm input; eul output
function eul = fcn(rotm)

    eul = rotm2eul(rotm,'ZYZ')

== matlab function NarwhaleSimscape/NarWhale/MATLAB Function3 ==
  data: q input; chi_dot output; qd input
function chi_dot  = FVK(q,qd)
q1 = q(1)
q2 = q(2)
q3 = q(3) 
q4 = q(4)
h1= 275.99/1000; % lasted
h2= 380/1000;
l1= 20/1000;
l2= 380/1000;
l3= 268.23/1000;
% q5 = q(5)
Je =[                                                                       0,                                                              -cos(q1),                                          -cos(q1),                     -cos(q1), sin(q2 + q3 + q4)*sin(q1);
                                                                           1,                                                                     0,                                                 0,                            0,        -cos(q2 + q3 + q4);
- sin(q1)*(l1 + l2*cos(q2 + q3) - h2*sin(q2)) - l3*sin(q2 + q3 + q4)*sin(q1), l3*cos(q2 + q3 + q4)*cos(q1) - cos(q1)*(l2*sin(q2 + q3) + h2*cos(q2)), -cos(q1)*(l2*sin(q2 + q3) - l3*cos(q2 + q3 + q4)), l3*cos(q2 + q3 + q4)*cos(q1),                         0;
  cos(q1)*(l1 + l2*cos(q2 + q3) - h2*sin(q2)) + l3*sin(q2 + q3 + q4)*cos(q1), l3*cos(q2 + q3 + q4)*sin(q1) - sin(q1)*(l2*sin(q2 + q3) + h2*cos(q2)), -sin(q1)*(l2*sin(q2 + q3) - l3*cos(q2 + q3 + q4)), l3*cos(q2 + q3 + q4)*sin(q1),                         0;
                                                                           0,                   l2*cos(q2 + q3) - h2*sin(q2) + l3*sin(q2 + q3 + q4),            l2*cos(q2 + q3) + l3*sin(q2 + q3 + q4),         l3*sin(q2 + q3 + q4),                         0]
chi_dot = Je * qd
end
